simulink model "pam_signal"  (R2025a)
settings: Solver=VariableStepAuto  StartTime=0.0  StopTime=10  RelTol=1e-3
settings Model: Creator=Bremdow  LastModifiedBy=Bremdow

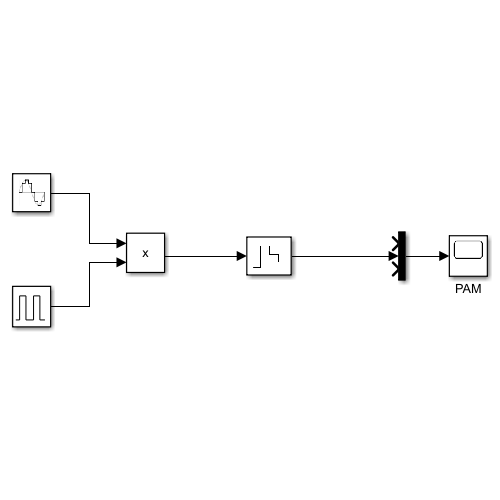
[thumbnail: Simulink's stored preview of the top-level diagram]
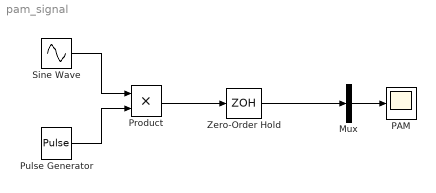
== system pam_signal ==
  Mux : Mux  Inputs=3
  PAM : Scope
      settings: ActiveDisplayYMinimum=-3.6159372666850877E-11  ActiveDisplayYMaximum=4.0177080740945413E-12  DataLoggingVariableName=pam_signal  DataLoggingSaveFormat=Array
  Product : Product
  Pulse Generator : DiscretePulseGenerator  PulseType=Time based  Period=0.0001
  Sine Wave : Sin  Amplitude=5  Frequency=2*pi*1000  SampleTime=1  VectorParams1D=off
  Zero-Order Hold : ZeroOrderHold  SampleTime=-1
  wires:
  Mux/1 -> PAM/1
  Sine Wave/1 -> Product/1
  Pulse Generator/1 -> Product/2
  Product/1 -> Zero-Order Hold/1
  Zero-Order Hold/1 -> Mux/2
